simulink model "heron_simulink"  (R2024a)
settings: Solver=VariableStepAuto  StartTime=0.0  StopTime=100  RelTol=1e-3
values from neighbouring files (symbols this model uses):
  A = 1    [heron.m]
  k = 1    [heron.m]    (also in oppg3_mekanikk.m)
  K = -1    [heron.m]
  r = 1    [heron.m]
  w = 0    [heron.m]
settings Model: Creator=filip  LastModifiedBy=filip

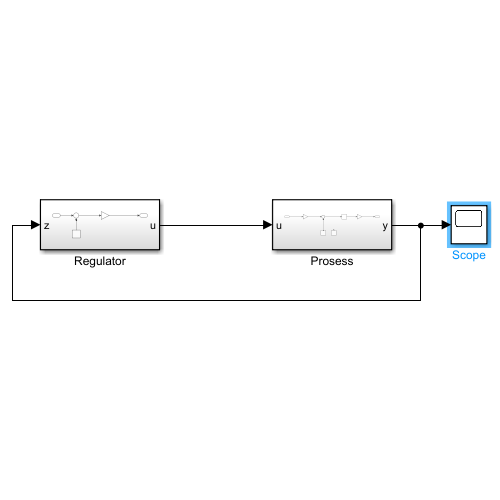
[thumbnail: Simulink's stored preview of the top-level diagram]
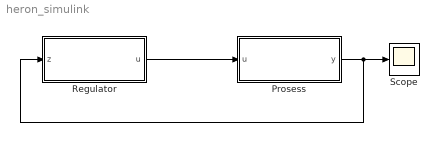
== system heron_simulink ==
  Prosess : Subsystem
  Regulator : Subsystem
  Scope : Scope
  wires:
  Regulator/1(u) -> Prosess/1(u)
  Prosess/1(y) -> Scope/1, Regulator/1(z)

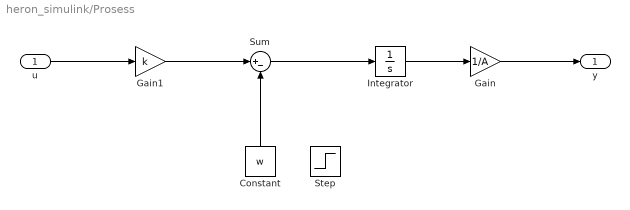
== system heron_simulink/Prosess ==
  u : Inport
  Constant : Constant  Value=w
  Gain : Gain  Gain=1/A
  Gain1 : Gain  Gain=k
  Integrator : Integrator  InitialCondition=0.5
  Step : Step  Time=10  After=0.1  SampleTime=0
  Sum : Sum  Inputs=|+-
  y : Outport
  wires:
  Integrator/1 -> Gain/1
  u/1 -> Gain1/1
  Gain1/1 -> Sum/1
  Sum/1 -> Integrator/1
  Gain/1 -> y/1
  Constant/1 -> Sum/2

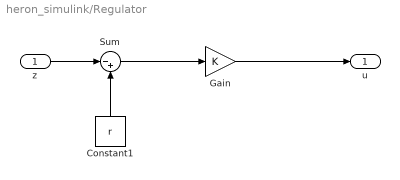
== system heron_simulink/Regulator ==
  z : Inport
  Constant1 : Constant  Value=r
  Gain : Gain  Gain=K
  Sum : Sum  Inputs=|-+
  u : Outport
  wires:
  z/1 -> Sum/1
  Constant1/1 -> Sum/2
  Sum/1 -> Gain/1
  Gain/1 -> u/1
